simulink model "Lab0_simulink"  (R2023a)
settings: Solver=VariableStepAuto  StartTime=0.0  StopTime=10.0  RelTol=1e-3
values from neighbouring files (symbols this model uses):
  a = 1 / (p + q)    (= 1)    [Lab0.m]
  b = r + w    (= 9)    [Lab0.m]
  c = p + q + r + w    (= 10)    [Lab0.m]
settings Model: Creator=user  LastModifiedBy=user

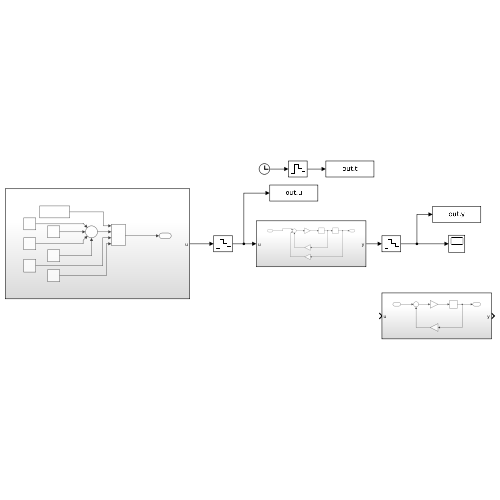
[thumbnail: Simulink's stored preview of the top-level diagram]
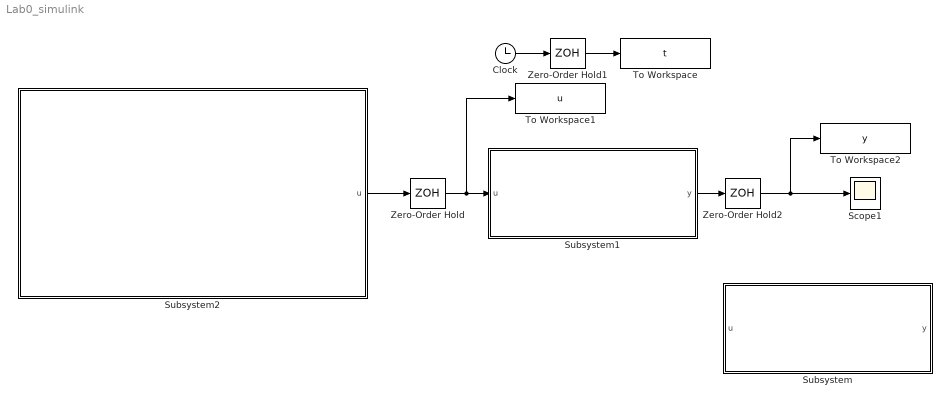
== system Lab0_simulink ==
  Clock : Clock
  Scope1 : Scope
  Subsystem : Subsystem
  Subsystem1 : Subsystem
  Subsystem2 : Subsystem
  To Workspace : ToWorkspace  VariableName=t  SampleTime=0.01
  To Workspace1 : ToWorkspace  VariableName=u  SampleTime=0.01
  To Workspace2 : ToWorkspace  VariableName=y  SampleTime=0.01
  Zero-Order Hold : ZeroOrderHold  SampleTime=0.01
  Zero-Order Hold1 : ZeroOrderHold  SampleTime=0.01
  Zero-Order Hold2 : ZeroOrderHold  SampleTime=0.01
  wires:
  Subsystem2/1(u) -> Zero-Order Hold/1
  Zero-Order Hold/1 -> Subsystem1/1(u), To Workspace1/1
  Clock/1 -> Zero-Order Hold1/1
  Zero-Order Hold1/1 -> To Workspace/1
  Subsystem1/1(y) -> Zero-Order Hold2/1
  Zero-Order Hold2/1 -> Scope1/1, To Workspace2/1

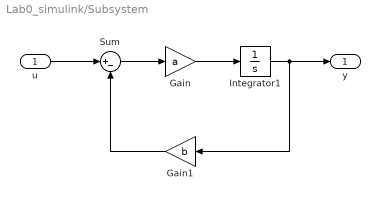
== system Lab0_simulink/Subsystem ==
  u : Inport
  Gain : Gain  Gain=a
  Gain1 : Gain  Gain=b
  Integrator1 : Integrator
  Sum : Sum  Inputs=|+-
  y : Outport
  wires:
  Gain/1 -> Integrator1/1
  Sum/1 -> Gain/1
  Gain1/1 -> Sum/2
  Integrator1/1 -> y/1, Gain1/1
  u/1 -> Sum/1

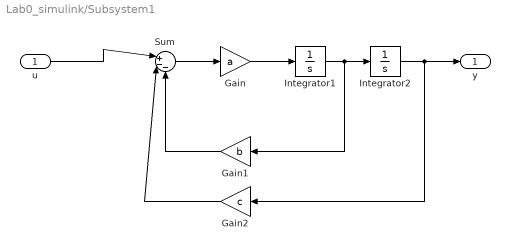
== system Lab0_simulink/Subsystem1 ==
  u : Inport
  Gain : Gain  Gain=a
  Gain1 : Gain  Gain=b
  Gain2 : Gain  Gain=c
  Integrator1 : Integrator
  Integrator2 : Integrator
  Sum : Sum  Inputs=|+--
  y : Outport
  wires:
  Sum/1 -> Gain/1
  Gain1/1 -> Sum/3
  Integrator1/1 -> Integrator2/1, Gain1/1
  Gain2/1 -> Sum/2
  Integrator2/1 -> y/1, Gain2/1
  Gain/1 -> Integrator1/1
  u/1 -> Sum/1

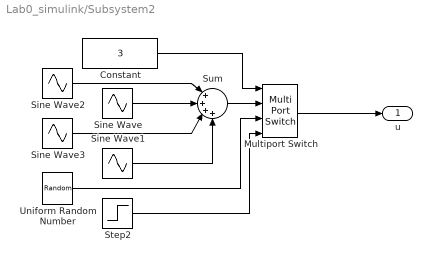
== system Lab0_simulink/Subsystem2 ==
  Constant : Constant  Value=3
  Multiport Switch : MultiPortSwitch  SaturateOnIntegerOverflow=off  InputSameDT=off
  Sine Wave : Sin  Amplitude=4  Frequency=8  SampleTime=0
  Sine Wave1 : Sin  Amplitude=4  Frequency=16  SampleTime=0
  Sine Wave2 : Sin  Amplitude=4  Frequency=4  SampleTime=0
  Sine Wave3 : Sin  Amplitude=4  Frequency=12  SampleTime=0
  Step2 : Step  After=2  SampleTime=0
  Sum : Sum  Inputs=|++++
  Uniform Random Number : UniformRandomNumber  Minimum=-4  Maximum=4  SampleTime=0.01
  u : Outport
  wires:
  Step2/1 -> Multiport Switch/4
  Sine Wave3/1 -> Sum/3
  Uniform Random Number/1 -> Multiport Switch/3
  Sum/1 -> Multiport Switch/2
  Multiport Switch/1 -> u/1
  Sine Wave1/1 -> Sum/4
  Sine Wave2/1 -> Sum/1
  Sine Wave/1 -> Sum/2
  Constant/1 -> Multiport Switch/1
